simulink model "MPC"  (R2017a)
settings: Solver=FixedStepAuto  StartTime=0.0  StopTime=10.0  FixedStep=1/60/10000  MaxStep=1e-4  RelTol=1e-3
undefined symbols (not defined in the file): R
libraries: powerlib x7, mpclib x1
settings Model: Creator=MarioAndres  LastModifiedBy=Administrador
settings OptimizationCC: DefaultParameterBehavior=Inlined  PassReuseOutputArgsAs=Individual arguments
settings DebuggingCC: ParameterTunabilityLossMsg=error
settings SFSimCC: MATLABDynamicMemAlloc=off
settings RTWCC: SystemTargetFile=ert.tlc  TemplateMakefile=ert_default_tmf  Description=Embedded Coder  GenerateReport=on  IncludeHyperlinkInReport=on  LaunchReport=on  GenerateTraceInfo=on  GenerateTraceReport=on  GenerateTraceReportSl=on  GenerateTraceReportSf=on  GenerateTraceReportEml=on
settings CodeAppCC: ForceParamTrailComments=on  IgnoreCustomStorageClasses=off  OperatorAnnotations=on  SimulinkDataObjDesc=on  SFDataObjDesc=on  MATLABFcnDesc=on  InsertBlockDesc=on  MATLABSourceComments=on
settings ERTTargetCC: TargetLangStandard=C99 (ISO)  GenerateSampleERTMain=on  InlinedParameterPlacement=NonHierarchical  ERTCustomFileTemplate=example_file_process.tlc

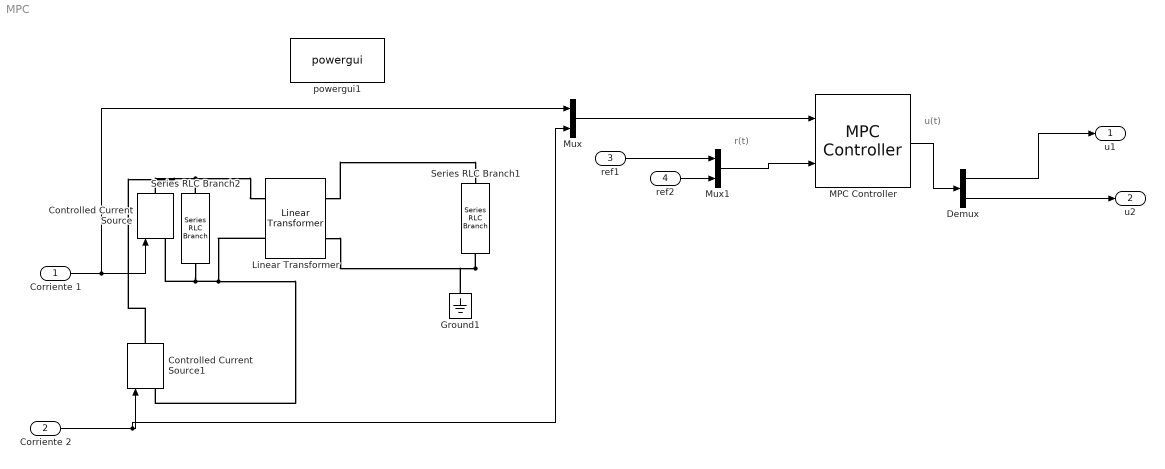
== system MPC ==
  note: u(t)
  note: r(t)
  Corriente 1 : Inport
  Corriente 2 : Inport  Port=2
  ref1 : Inport  Port=3
  ref2 : Inport  Port=4
  Controlled Current Source : powerlib/Electrical Sources/Controlled Current Source  Initialize=on  Source_Type=AC  Amplitude=0  Phase=0  Frequency=0  Measurements=None
  Controlled Current Source1 : powerlib/Electrical Sources/Controlled Current Source  Initialize=on  Source_Type=AC  Amplitude=0  Phase=0  Frequency=0  Measurements=None
  Demux : Demux  Outputs=2
  Ground1 : powerlib/Elements/Ground  LConnTagsString=a
  Linear Transformer : powerlib/Elements/Linear Transformer  UNITS=SI  NominalPower=[ 1500 60 ]  winding1=[141.2 0 0.003]  winding2=[120 0.004 0.084225]  ThreeWindings=off  winding3=[3.15e+05 0.7938 0.084225]  RmLm=[1.0805e+06 2866]  Measurements=None  DataType=on
  MPC Controller : mpclib/MPC Controller  mpcobj=mpcobj  x0=[]  is_multiple=0  enable_value=0  return_u0=off  ref_from_ws=off  ref_signal_name=[]  ref_preview=on  md_from_ws=off  md_signal_name=[]  md_preview=on  from_project=off  project_file=MPCtask.mat  md_inport=off  mv_inport=off  cost_outport=off  return_sequence=off  return_qpstatus=off  return_state=off  state_inport=off  lims_inport=off  ywt_inport=off  is_designfromscratch=0  uwt_inport=off  duwt_inport=off  rhoeps_inport=off  uref_inport=off  n_ts=0.1  n_mv=2  n_md=0  n_ud=0  n_mo=2  n_uo=0  BlockDataType=double  SampleTimeInherited=off  switch_inport=off
  Mux : Mux  Inputs=2
  Mux1 : Mux  Inputs=2
  Series RLC Branch1 : powerlib/Elements/Series RLC Branch  LConnTagsString=__new0  RConnTagsString=__new0  BranchType=R  Resistance=R  Inductance=25e-3  SetiL0=off  InitialCurrent=0  Capacitance=5.30e-3  Setx0=off  InitialVoltage=0  Measurements=None
  Series RLC Branch2 : powerlib/Elements/Series RLC Branch  LConnTagsString=__new0  RConnTagsString=__new0  BranchType=R  Resistance=100000000  Inductance=25e-3  SetiL0=off  InitialCurrent=0  Capacitance=5.30e-3  Setx0=off  InitialVoltage=0  Measurements=None
  powergui1 : powerlib/powergui  SimulationMode=Discrete  SampleTime=1/60/10000  frequency=60  Iterations=50  frequencyindice=0  Pbase=100e6  ErrMax=1e-4  UnitsV=kV  UnitsW=MW  buscounter=0  FunctionMessages=off  echomessages=off  EnableUseOfTLC=off  CurrentSourceSwitches=off  DisableSnubberDevices=off  DisableRonSwitches=off  DisableVfSwitches=off  DisplayEquations=off  SolverType=Tustin/Backward Euler (TBE)  Interpol=off  ExternalGateDelay=off  methode=off  Ts=100  x0status=blocks  SPID=off  SwTol=0  HookPort=off  RestoreLinks=warning  ResistiveCurrentMeasurement=off  Frange=[0:2:500]  Ylog=off  Xlog=on  ShowGrid=off  save=off  variable=ZData  structure=sps1phPWM1_str  ZoomFFT=on  StartTime=0.1-2/60  cycles=2  DisplayStyle=1  fundamental=60  FreqAxis=off  MaxFrequency=5000  frequencyindicesteady=1  RmsSteady=1  display=off
  u1 : Outport
  u2 : Outport  Port=2
  wires:
  Corriente 1/1 -> Controlled Current Source/1, Mux/1
  Demux/2 -> u2/1
  Mux1/1 -> MPC Controller/2
  MPC Controller/1 -> Demux/1
  Demux/1 -> u1/1
  Corriente 2/1 -> Controlled Current Source1/1, Mux/2
  Mux/1 -> MPC Controller/1
  ref1/1 -> Mux1/1
  ref2/1 -> Mux1/2
  connections:
  Linear Transformer/RConn1 -- Series RLC Branch1/LConn1
  Series RLC Branch1/RConn1 -- Ground1/LConn1 -- Linear Transformer/RConn2
  Controlled Current Source1/RConn1 -- Controlled Current Source/RConn1 -- Series RLC Branch2/LConn1 -- Linear Transformer/LConn1
  Linear Transformer/LConn2 -- Controlled Current Source1/LConn1 -- Series RLC Branch2/RConn1 -- Controlled Current Source/LConn1
